simulink library "ammclib_bam_S32K14x"  (R2016a)
settings: Solver=VariableStepAuto  SolverMode=SingleTasking  StartTime=0.0  StopTime=10.0  RelTol=1e-3
undefined symbols (not defined in the file or in its folder): f16A1, f16A2, f16ADCMaxError, f16B0, f16B1, f16B2, f16C1, f16CC1, f16CC1sc, f16CC1sc_D, f16CC1sc_Q, f16CC2, f16CC2sc, f16CC2sc_D, f16CC2sc_Q, f16DerivGain, f16EGain, f16FiltCoef, f16HystOff, f16HystOn, f16IGain, f16IntegGain, f16IntegGainFW, f16IntegGainQ, f16Kd, f16Kq, f16Limit, f16LowerLimit, f16LowerLimit_D, f16LowerLimit_Q, f16LowerLimitFW, f16LowerLimitQ, f16ModIndex, f16OutValOff, f16OutValOn, f16PropGain, f16PropGainFW, f16PropGainQ, f16RampDown, f16RampUp, f16UGain, f16UpperLimit, f16UpperLimit_D, f16UpperLimit_Q, f16UpperLimitFW, f16UpperLimitQ, f16WIGain, f32A1, f32A2, f32ADCMaxError, f32B0, f32B1, f32B2, f32C1, f32CC1, f32CC1sc, f32CC1sc_D, f32CC1sc_Q, f32CC2, f32CC2sc ... (+114)
(part 18 of 22)

== system ammclib_bam_S32K14x/AMCLIB/FLT/AMCLIB_Windmilling_FLT ==
  pUabcIn : Inport  OutDataTypeStr=Bus: SWLIBS_3Syst_FLT  BusOutputAsStruct=on
  AMCLIB_Windmilling_SF : S-Function  FunctionName=AMCLIB_Windmilling_SF_FLT  Parameters=showStates,fltADCMaxError,fltCC1sc,fltCC2sc,fltUpperLimit,fltLowerLimit,fltC1  SFunctionDeploymentMode=off  EnableBusSupport=off
  copyright : Subsystem
      mask Display: text(10,90,'FILE:');text(10,75,'DESRIPTION:');text(10,60,'COPYRIGHT:');text(10,45,'VERSION:');text(10,30,'DATE:')
  copyright2 : Subsystem
      mask Display: text(10,90,'AMCLIB_Windmilling_BAM_FLT.mdl');text(10,75,'PMSM Windmilling');text(10,60,'NXP 2020');text(10,45,'1.0');text(10,30,'28-Mar-2020');
  fltADCMaxError : Ground
  fltAccPI : Ground
  fltAccPI_Out : Terminator
  fltC1 : Ground
  fltCC1sc : Ground
  fltCC2sc : Ground
  fltInErrK1 : Ground
  fltInErrK1_Out : Terminator
  fltInK1 : Ground
  fltInK1_Out : Terminator
  fltLowerLimit : Ground
  fltState : Ground
  fltState_Out : Terminator
  fltUpperLimit : Ground
  u32Lock : Outport
  pPosEst : Outport  Port=2
  pVelocityEst : Outport  Port=3
  wires:
  AMCLIB_Windmilling_SF/7 -> fltInK1_Out/1
  AMCLIB_Windmilling_SF/6 -> fltState_Out/1
  AMCLIB_Windmilling_SF/5 -> fltInErrK1_Out/1
  AMCLIB_Windmilling_SF/4 -> fltAccPI_Out/1
  AMCLIB_Windmilling_SF/3 -> pVelocityEst/1
  AMCLIB_Windmilling_SF/2 -> pPosEst/1
  AMCLIB_Windmilling_SF/1 -> u32Lock/1
  fltInK1/1 -> AMCLIB_Windmilling_SF/11
  fltState/1 -> AMCLIB_Windmilling_SF/10
  fltInErrK1/1 -> AMCLIB_Windmilling_SF/9
  fltAccPI/1 -> AMCLIB_Windmilling_SF/8
  fltC1/1 -> AMCLIB_Windmilling_SF/7
  fltLowerLimit/1 -> AMCLIB_Windmilling_SF/6
  fltUpperLimit/1 -> AMCLIB_Windmilling_SF/5
  fltCC2sc/1 -> AMCLIB_Windmilling_SF/4
  fltCC1sc/1 -> AMCLIB_Windmilling_SF/3
  fltADCMaxError/1 -> AMCLIB_Windmilling_SF/2
  pUabcIn/1 -> AMCLIB_Windmilling_SF/1

== system ammclib_bam_S32K14x/GDFLIB/F16/GDFLIB_FilterFIR_F16 ==
  f16In : Inport  OutDataTypeStr=int16
  GDFLIB_FilterFIR_SF : S-Function  FunctionName=GDFLIB_FilterFIR_SF_F16  Parameters=u16Order,pCoefBuf  SFunctionDeploymentMode=off  EnableBusSupport=off
  copyright : Subsystem
      mask Display: text(10,90,'FILE:');text(10,75,'DESRIPTION:');text(10,60,'COPYRIGHT:');text(10,45,'VERSION:');text(10,30,'DATE:')
  copyright2 : Subsystem
      mask Display: text(10,90,'GDFLIB_FilterFIR_BAM_F16.mdl');text(10,75,'FIR filter.');text(10,60,'NXP 2020');text(10,45,'1.0');text(10,30,'18-Mar-2020');
  f16Out : Outport
  wires:
  GDFLIB_FilterFIR_SF/1 -> f16Out/1
  f16In/1 -> GDFLIB_FilterFIR_SF/1

== system ammclib_bam_S32K14x/GDFLIB/F16/GDFLIB_FilterIIR1_F16 ==
  f16In : Inport  OutDataTypeStr=int16
  GDFLIB_FilterIIR1_SF : S-Function  FunctionName=GDFLIB_FilterIIR1_SF_F16  Parameters=showStates,f16B0,f16B1,f16A1  SFunctionDeploymentMode=off  EnableBusSupport=off
  copyright : Subsystem
      mask Display: text(10,90,'FILE:');text(10,75,'DESRIPTION:');text(10,60,'COPYRIGHT:');text(10,45,'VERSION:');text(10,30,'DATE:')
  copyright2 : Subsystem
      mask Display: text(10,90,'GDFLIB_FilterIIR1_BAM_F16.mdl');text(10,75,'First order IIR filter.');text(10,60,'NXP 2020');text(10,45,'1.0');text(10,30,'18-Mar-2020');
  f16A1 : Ground
  f16B0 : Ground
  f16B1 : Ground
  f16FiltBufferX : Ground
  f16FiltBufferX_Out : Terminator
  f32FiltBufferY : Ground
  f32FiltBufferY_Out : Terminator
  f16Out : Outport
  wires:
  GDFLIB_FilterIIR1_SF/3 -> f32FiltBufferY_Out/1
  GDFLIB_FilterIIR1_SF/2 -> f16FiltBufferX_Out/1
  GDFLIB_FilterIIR1_SF/1 -> f16Out/1
  f32FiltBufferY/1 -> GDFLIB_FilterIIR1_SF/6
  f16FiltBufferX/1 -> GDFLIB_FilterIIR1_SF/5
  f16A1/1 -> GDFLIB_FilterIIR1_SF/4
  f16B1/1 -> GDFLIB_FilterIIR1_SF/3
  f16B0/1 -> GDFLIB_FilterIIR1_SF/2
  f16In/1 -> GDFLIB_FilterIIR1_SF/1

== system ammclib_bam_S32K14x/GDFLIB/F16/GDFLIB_FilterIIR2_F16 ==
  f16In : Inport  OutDataTypeStr=int16
  FilterBufferX1_Out : Terminator
  FilterBufferX2_Out : Terminator
  FilterBufferY1_Out : Terminator
  FilterBufferY2_Out : Terminator
  GDFLIB_FilterIIR2_SF : S-Function  FunctionName=GDFLIB_FilterIIR2_SF_F16  Parameters=showStates,f16B0,f16B1,f16B2,f16A1,f16A2  SFunctionDeploymentMode=off  EnableBusSupport=off
  copyright : Subsystem
      mask Display: text(10,90,'FILE:');text(10,75,'DESRIPTION:');text(10,60,'COPYRIGHT:');text(10,45,'VERSION:');text(10,30,'DATE:')
  copyright2 : Subsystem
      mask Display: text(10,90,'GDFLIB_FilterIIR2_BAM_F16.mdl');text(10,75,'First order IIR filter.');text(10,60,'NXP 2020');text(10,45,'1.0');text(10,30,'18-Mar-2020');
  f16A1 : Ground
  f16A2 : Ground
  f16B0 : Ground
  f16B1 : Ground
  f16B2 : Ground
  f16FiltBufferX1 : Ground
  f16FiltBufferX2 : Ground
  f32FiltBufferY1 : Ground
  f32FiltBufferY2 : Ground
  f16Out : Outport
  wires:
  GDFLIB_FilterIIR2_SF/5 -> FilterBufferY2_Out/1
  GDFLIB_FilterIIR2_SF/4 -> FilterBufferY1_Out/1
  GDFLIB_FilterIIR2_SF/3 -> FilterBufferX2_Out/1
  GDFLIB_FilterIIR2_SF/2 -> FilterBufferX1_Out/1
  GDFLIB_FilterIIR2_SF/1 -> f16Out/1
  f16A2/1 -> GDFLIB_FilterIIR2_SF/10
  f16A1/1 -> GDFLIB_FilterIIR2_SF/9
  f16B2/1 -> GDFLIB_FilterIIR2_SF/8
  f16B1/1 -> GDFLIB_FilterIIR2_SF/7
  f16B0/1 -> GDFLIB_FilterIIR2_SF/6
  f32FiltBufferY2/1 -> GDFLIB_FilterIIR2_SF/5
  f32FiltBufferY1/1 -> GDFLIB_FilterIIR2_SF/4
  f16FiltBufferX2/1 -> GDFLIB_FilterIIR2_SF/3
  f16FiltBufferX1/1 -> GDFLIB_FilterIIR2_SF/2
  f16In/1 -> GDFLIB_FilterIIR2_SF/1

== system ammclib_bam_S32K14x/GDFLIB/F16/GDFLIB_FilterMA_F16 ==
  f16In : Inport  OutDataTypeStr=int16
  f16FilterMAOut_preset : Inport  Port=2  OutDataTypeStr=int16
  Reset : ResetPort  DisableCoverage=on
  GDFLIB_FilterMA_SF : S-Function  FunctionName=GDFLIB_FilterMA_SF_F16  Parameters=showStates,resetStatesEnable,u16NSamples  SFunctionDeploymentMode=off  EnableBusSupport=off
  copyright : Subsystem
      mask Display: text(10,90,'FILE:');text(10,75,'DESRIPTION:');text(10,60,'COPYRIGHT:');text(10,45,'VERSION:');text(10,30,'DATE:')
  copyright2 : Subsystem
      mask Display: text(10,90,'GDFLIB_FilterMA_BAM_F16.mdl');text(10,75,'Exponential moving average filter.');text(10,60,'NXP 2020');text(10,45,'1.0');text(10,30,'28-Mar-2020');
  f32Acc : Ground
  f32Acc_Out : Terminator
  u16NSamples : Ground
  f16Out : Outport
  wires:
  GDFLIB_FilterMA_SF/2 -> f32Acc_Out/1
  GDFLIB_FilterMA_SF/1 -> f16Out/1
  f32Acc/1 -> GDFLIB_FilterMA_SF/4
  u16NSamples/1 -> GDFLIB_FilterMA_SF/3
  f16FilterMAOut_preset/1 -> GDFLIB_FilterMA_SF/2
  f16In/1 -> GDFLIB_FilterMA_SF/1

== system ammclib_bam_S32K14x/GDFLIB/F32/GDFLIB_FilterFIR_F32 ==
  f32In : Inport  OutDataTypeStr=int32
  GDFLIB_FilterFIR_SF : S-Function  FunctionName=GDFLIB_FilterFIR_SF_F32  Parameters=u32Order,pCoefBuf  SFunctionDeploymentMode=off  EnableBusSupport=off
  copyright : Subsystem
      mask Display: text(10,90,'FILE:');text(10,75,'DESRIPTION:');text(10,60,'COPYRIGHT:');text(10,45,'VERSION:');text(10,30,'DATE:')
  copyright2 : Subsystem
      mask Display: text(10,90,'GDFLIB_FilterFIR_BAM_F32.mdl');text(10,75,'FIR filter.');text(10,60,'NXP 2020');text(10,45,'1.0');text(10,30,'18-Mar-2020');
  f32Out : Outport
  wires:
  GDFLIB_FilterFIR_SF/1 -> f32Out/1
  f32In/1 -> GDFLIB_FilterFIR_SF/1

== system ammclib_bam_S32K14x/GDFLIB/F32/GDFLIB_FilterIIR1_F32 ==
  f32In : Inport  OutDataTypeStr=int32
  GDFLIB_FilterIIR1_SF : S-Function  FunctionName=GDFLIB_FilterIIR1_SF_F32  Parameters=showStates,f32B0,f32B1,f32A1  SFunctionDeploymentMode=off  EnableBusSupport=off
  copyright : Subsystem
      mask Display: text(10,90,'FILE:');text(10,75,'DESRIPTION:');text(10,60,'COPYRIGHT:');text(10,45,'VERSION:');text(10,30,'DATE:')
  copyright2 : Subsystem
      mask Display: text(10,90,'GDFLIB_FilterIIR1_BAM_F32.mdl');text(10,75,'First order IIR filter.');text(10,60,'NXP 2020');text(10,45,'1.0');text(10,30,'18-Mar-2020');
  f32A1 : Ground
  f32B0 : Ground
  f32B1 : Ground
  f32FiltBufferX : Ground
  f32FiltBufferX_Out : Terminator
  f32FiltBufferY : Ground
  f32FiltBufferY_Out : Terminator
  f32Out : Outport
  wires:
  GDFLIB_FilterIIR1_SF/3 -> f32FiltBufferY_Out/1
  GDFLIB_FilterIIR1_SF/2 -> f32FiltBufferX_Out/1
  GDFLIB_FilterIIR1_SF/1 -> f32Out/1
  f32FiltBufferY/1 -> GDFLIB_FilterIIR1_SF/6
  f32FiltBufferX/1 -> GDFLIB_FilterIIR1_SF/5
  f32A1/1 -> GDFLIB_FilterIIR1_SF/4
  f32B1/1 -> GDFLIB_FilterIIR1_SF/3
  f32B0/1 -> GDFLIB_FilterIIR1_SF/2
  f32In/1 -> GDFLIB_FilterIIR1_SF/1

== system ammclib_bam_S32K14x/GDFLIB/F32/GDFLIB_FilterIIR2_F32 ==
  f32In : Inport  OutDataTypeStr=int32
  FilterBufferX1_Out : Terminator
  FilterBufferX2_Out : Terminator
  FilterBufferY1_Out : Terminator
  FilterBufferY2_Out : Terminator
  GDFLIB_FilterIIR2_SF : S-Function  FunctionName=GDFLIB_FilterIIR2_SF_F32  Parameters=showStates,f32B0,f32B1,f32B2,f32A1,f32A2  SFunctionDeploymentMode=off  EnableBusSupport=off
  copyright : Subsystem
      mask Display: text(10,90,'FILE:');text(10,75,'DESRIPTION:');text(10,60,'COPYRIGHT:');text(10,45,'VERSION:');text(10,30,'DATE:')
  copyright2 : Subsystem
      mask Display: text(10,90,'GDFLIB_FilterIIR2_BAM_F32.mdl');text(10,75,'First order IIR filter.');text(10,60,'NXP 2020');text(10,45,'1.0');text(10,30,'18-Mar-2020');
  f32A1 : Ground
  f32A2 : Ground
  f32B0 : Ground
  f32B1 : Ground
  f32B2 : Ground
  f32FiltBufferX1 : Ground
  f32FiltBufferX2 : Ground
  f32FiltBufferY1 : Ground
  f32FiltBufferY2 : Ground
  f32Out : Outport
  wires:
  GDFLIB_FilterIIR2_SF/5 -> FilterBufferY2_Out/1
  GDFLIB_FilterIIR2_SF/4 -> FilterBufferY1_Out/1
  GDFLIB_FilterIIR2_SF/3 -> FilterBufferX2_Out/1
  GDFLIB_FilterIIR2_SF/2 -> FilterBufferX1_Out/1
  GDFLIB_FilterIIR2_SF/1 -> f32Out/1
  f32A2/1 -> GDFLIB_FilterIIR2_SF/10
  f32A1/1 -> GDFLIB_FilterIIR2_SF/9
  f32B2/1 -> GDFLIB_FilterIIR2_SF/8
  f32B1/1 -> GDFLIB_FilterIIR2_SF/7
  f32B0/1 -> GDFLIB_FilterIIR2_SF/6
  f32FiltBufferY2/1 -> GDFLIB_FilterIIR2_SF/5
  f32FiltBufferY1/1 -> GDFLIB_FilterIIR2_SF/4
  f32FiltBufferX2/1 -> GDFLIB_FilterIIR2_SF/3
  f32FiltBufferX1/1 -> GDFLIB_FilterIIR2_SF/2
  f32In/1 -> GDFLIB_FilterIIR2_SF/1

== system ammclib_bam_S32K14x/GDFLIB/F32/GDFLIB_FilterMA_F32 ==
  f32In : Inport  OutDataTypeStr=int32
  f32FilterMAOut_preset : Inport  Port=2  OutDataTypeStr=int32
  Reset : ResetPort  DisableCoverage=on
  GDFLIB_FilterMA_SF : S-Function  FunctionName=GDFLIB_FilterMA_SF_F32  Parameters=showStates,resetStatesEnable,u16NSamples  SFunctionDeploymentMode=off  EnableBusSupport=off
  copyright : Subsystem
      mask Display: text(10,90,'FILE:');text(10,75,'DESRIPTION:');text(10,60,'COPYRIGHT:');text(10,45,'VERSION:');text(10,30,'DATE:')
  copyright2 : Subsystem
      mask Display: text(10,90,'GDFLIB_FilterMA_BAM_F32.mdl');text(10,75,'Exponential moving average filter.');text(10,60,'NXP 2020');text(10,45,'1.0');text(10,30,'28-Mar-2020');
  f32Acc : Ground
  f32Acc_Out : Terminator
  u16NSamples : Ground
  f32Out : Outport
  wires:
  GDFLIB_FilterMA_SF/2 -> f32Acc_Out/1
  GDFLIB_FilterMA_SF/1 -> f32Out/1
  f32Acc/1 -> GDFLIB_FilterMA_SF/4
  u16NSamples/1 -> GDFLIB_FilterMA_SF/3
  f32FilterMAOut_preset/1 -> GDFLIB_FilterMA_SF/2
  f32In/1 -> GDFLIB_FilterMA_SF/1

== system ammclib_bam_S32K14x/GDFLIB/FLT/GDFLIB_FilterFIR_FLT ==
  fltIn : Inport  OutDataTypeStr=single
  GDFLIB_FilterFIR_SF : S-Function  FunctionName=GDFLIB_FilterFIR_SF_FLT  Parameters=u32Order,pCoefBuf  SFunctionDeploymentMode=off  EnableBusSupport=off
  copyright : Subsystem
      mask Display: text(10,90,'FILE:');text(10,75,'DESRIPTION:');text(10,60,'COPYRIGHT:');text(10,45,'VERSION:');text(10,30,'DATE:')
  copyright2 : Subsystem
      mask Display: text(10,90,'GDFLIB_FilterFIR_BAM_FLT.mdl');text(10,75,'FIR filter.');text(10,60,'NXP 2020');text(10,45,'1.0');text(10,30,'18-Mar-2020');
  fltOut : Outport
  wires:
  GDFLIB_FilterFIR_SF/1 -> fltOut/1
  fltIn/1 -> GDFLIB_FilterFIR_SF/1

== system ammclib_bam_S32K14x/GDFLIB/FLT/GDFLIB_FilterIIR1_FLT ==
  fltIn : Inport  OutDataTypeStr=single
  GDFLIB_FilterIIR1_SF : S-Function  FunctionName=GDFLIB_FilterIIR1_SF_FLT  Parameters=showStates,fltB0,fltB1,fltA1  SFunctionDeploymentMode=off  EnableBusSupport=off
  copyright : Subsystem
      mask Display: text(10,90,'FILE:');text(10,75,'DESRIPTION:');text(10,60,'COPYRIGHT:');text(10,45,'VERSION:');text(10,30,'DATE:')
  copyright2 : Subsystem
      mask Display: text(10,90,'GDFLIB_FilterIIR1_BAM_FLT.mdl');text(10,75,'First order IIR filter.');text(10,60,'NXP 2020');text(10,45,'1.0');text(10,30,'18-Mar-2020');
  fltA1 : Ground
  fltB0 : Ground
  fltB1 : Ground
  fltFiltBufferX : Ground
  fltFiltBufferX_Out : Terminator
  fltFiltBufferY : Ground
  fltFiltBufferY_Out : Terminator
  fltOut : Outport
  wires:
  GDFLIB_FilterIIR1_SF/3 -> fltFiltBufferY_Out/1
  GDFLIB_FilterIIR1_SF/2 -> fltFiltBufferX_Out/1
  GDFLIB_FilterIIR1_SF/1 -> fltOut/1
  fltFiltBufferY/1 -> GDFLIB_FilterIIR1_SF/6
  fltFiltBufferX/1 -> GDFLIB_FilterIIR1_SF/5
  fltA1/1 -> GDFLIB_FilterIIR1_SF/4
  fltB1/1 -> GDFLIB_FilterIIR1_SF/3
  fltB0/1 -> GDFLIB_FilterIIR1_SF/2
  fltIn/1 -> GDFLIB_FilterIIR1_SF/1

== system ammclib_bam_S32K14x/GDFLIB/FLT/GDFLIB_FilterIIR2_FLT ==
  fltIn : Inport  OutDataTypeStr=single
  FilterBufferX1_Out : Terminator
  FilterBufferX2_Out : Terminator
  FilterBufferY1_Out : Terminator
  FilterBufferY2_Out : Terminator
  GDFLIB_FilterIIR2_SF : S-Function  FunctionName=GDFLIB_FilterIIR2_SF_FLT  Parameters=showStates,fltB0,fltB1,fltB2,fltA1,fltA2  SFunctionDeploymentMode=off  EnableBusSupport=off
  copyright : Subsystem
      mask Display: text(10,90,'FILE:');text(10,75,'DESRIPTION:');text(10,60,'COPYRIGHT:');text(10,45,'VERSION:');text(10,30,'DATE:')
  copyright2 : Subsystem
      mask Display: text(10,90,'GDFLIB_FilterIIR2_BAM_FLT.mdl');text(10,75,'First order IIR filter.');text(10,60,'NXP 2020');text(10,45,'1.0');text(10,30,'18-Mar-2020');
  fltA1 : Ground
  fltA2 : Ground
  fltB0 : Ground
  fltB1 : Ground
  fltB2 : Ground
  fltFiltBufferX1 : Ground
  fltFiltBufferX2 : Ground
  fltFiltBufferY1 : Ground
  fltFiltBufferY2 : Ground
  fltOut : Outport
  wires:
  GDFLIB_FilterIIR2_SF/5 -> FilterBufferY2_Out/1
  GDFLIB_FilterIIR2_SF/4 -> FilterBufferY1_Out/1
  GDFLIB_FilterIIR2_SF/3 -> FilterBufferX2_Out/1
  GDFLIB_FilterIIR2_SF/2 -> FilterBufferX1_Out/1
  GDFLIB_FilterIIR2_SF/1 -> fltOut/1
  fltA2/1 -> GDFLIB_FilterIIR2_SF/10
  fltA1/1 -> GDFLIB_FilterIIR2_SF/9
  fltB2/1 -> GDFLIB_FilterIIR2_SF/8
  fltB1/1 -> GDFLIB_FilterIIR2_SF/7
  fltB0/1 -> GDFLIB_FilterIIR2_SF/6
  fltFiltBufferY2/1 -> GDFLIB_FilterIIR2_SF/5
  fltFiltBufferY1/1 -> GDFLIB_FilterIIR2_SF/4
  fltFiltBufferX2/1 -> GDFLIB_FilterIIR2_SF/3
  fltFiltBufferX1/1 -> GDFLIB_FilterIIR2_SF/2
  fltIn/1 -> GDFLIB_FilterIIR2_SF/1

== system ammclib_bam_S32K14x/GDFLIB/FLT/GDFLIB_FilterMA_FLT ==
  fltIn : Inport  OutDataTypeStr=single
  fltFilterMAOut_preset : Inport  Port=2  OutDataTypeStr=single
  Reset : ResetPort  DisableCoverage=on
  GDFLIB_FilterMA_SF : S-Function  FunctionName=GDFLIB_FilterMA_SF_FLT  Parameters=showStates,resetStatesEnable,fltLambda  SFunctionDeploymentMode=off  EnableBusSupport=off
  copyright : Subsystem
      mask Display: text(10,90,'FILE:');text(10,75,'DESRIPTION:');text(10,60,'COPYRIGHT:');text(10,45,'VERSION:');text(10,30,'DATE:')
  copyright2 : Subsystem
      mask Display: text(10,90,'GDFLIB_FilterMA_BAM_FLT.mdl');text(10,75,'Exponential moving average filter.');text(10,60,'NXP 2020');text(10,45,'1.0');text(10,30,'28-Mar-2020');
  fltAcc : Ground
  fltAcc_Out : Terminator
  fltLambda : Ground
  fltOut : Outport
  wires:
  GDFLIB_FilterMA_SF/2 -> fltAcc_Out/1
  GDFLIB_FilterMA_SF/1 -> fltOut/1
  fltAcc/1 -> GDFLIB_FilterMA_SF/4
  fltLambda/1 -> GDFLIB_FilterMA_SF/3
  fltFilterMAOut_preset/1 -> GDFLIB_FilterMA_SF/2
  fltIn/1 -> GDFLIB_FilterMA_SF/1

== system ammclib_bam_S32K14x/GFLIB/F16/GFLIB_Acos_F16 ==
  f16In : Inport  OutDataTypeStr=int16
  GFLIB_Acos_SF : S-Function  FunctionName=GFLIB_Acos_SF_F16  SFunctionDeploymentMode=off  EnableBusSupport=off
  copyright : Subsystem
      mask Display: text(10,90,'FILE:');text(10,75,'DESRIPTION:');text(10,60,'COPYRIGHT:');text(10,45,'VERSION:');text(10,30,'DATE:')
  copyright2 : Subsystem
      mask Display: text(10,90,'GFLIB_Acos_BAM_F16.mdl');text(10,75,'Inverse cosine function');text(10,60,'NXP 2020');text(10,45,'1.0');text(10,30,'18-Mar-2020');
  f16Out : Outport
  wires:
  GFLIB_Acos_SF/1 -> f16Out/1
  f16In/1 -> GFLIB_Acos_SF/1

== system ammclib_bam_S32K14x/GFLIB/F16/GFLIB_Asin_F16 ==
  f16In : Inport  OutDataTypeStr=int16
  GFLIB_Asin_SF : S-Function  FunctionName=GFLIB_Asin_SF_F16  SFunctionDeploymentMode=off  EnableBusSupport=off
  copyright : Subsystem
      mask Display: text(10,90,'FILE:');text(10,75,'DESRIPTION:');text(10,60,'COPYRIGHT:');text(10,45,'VERSION:');text(10,30,'DATE:')
  copyright2 : Subsystem
      mask Display: text(10,90,'GFLIB_Asin_BAM_F16.mdl');text(10,75,'Inverse sine function');text(10,60,'NXP 2020');text(10,45,'1.0');text(10,30,'18-Mar-2020');
  f16Out : Outport
  wires:
  GFLIB_Asin_SF/1 -> f16Out/1
  f16In/1 -> GFLIB_Asin_SF/1

== system ammclib_bam_S32K14x/GFLIB/F16/GFLIB_AtanYXShifted_F16 ==
  f16InY : Inport  OutDataTypeStr=int16
  f16InX : Inport  Port=2  OutDataTypeStr=int16
  Ky : Inport  Port=3  OutDataTypeStr=int16
  Kx : Inport  Port=4  OutDataTypeStr=int16
  Ny : Inport  Port=5  OutDataTypeStr=int16
  Nx : Inport  Port=6  OutDataTypeStr=int16
  ThetaAdj : Inport  Port=7  OutDataTypeStr=int16
  GFLIB_AtanYXShifted_SF : S-Function  FunctionName=GFLIB_AtanYXShifted_SF_F16  SFunctionDeploymentMode=off  EnableBusSupport=off
  copyright : Subsystem
      mask Display: text(10,90,'FILE:');text(10,75,'DESRIPTION:');text(10,60,'COPYRIGHT:');text(10,45,'VERSION:');text(10,30,'DATE:')
  copyright2 : Subsystem
      mask Display: text(10,90,'GFLIB_AtanYXShifted_BAM_F16.mdl');text(10,75,'Shifted arctangent of two arguments Y/X.');text(10,60,'NXP 2020');text(10,45,'1.0');text(10,30,'18-Mar-2020');
  f16Out : Outport
  wires:
  GFLIB_AtanYXShifted_SF/1 -> f16Out/1
  ThetaAdj/1 -> GFLIB_AtanYXShifted_SF/7
  Nx/1 -> GFLIB_AtanYXShifted_SF/6
  Ny/1 -> GFLIB_AtanYXShifted_SF/5
  Kx/1 -> GFLIB_AtanYXShifted_SF/4
  Ky/1 -> GFLIB_AtanYXShifted_SF/3
  f16InX/1 -> GFLIB_AtanYXShifted_SF/2
  f16InY/1 -> GFLIB_AtanYXShifted_SF/1

== system ammclib_bam_S32K14x/GFLIB/F16/GFLIB_AtanYX_F16 ==
  f16InY : Inport  OutDataTypeStr=int16
  f16InX : Inport  Port=2  OutDataTypeStr=int16
  GFLIB_AtanYX_SF : S-Function  FunctionName=GFLIB_AtanYX_SF_F16  SFunctionDeploymentMode=off  EnableBusSupport=off
  copyright : Subsystem
      mask Display: text(10,90,'FILE:');text(10,75,'DESRIPTION:');text(10,60,'COPYRIGHT:');text(10,45,'VERSION:');text(10,30,'DATE:')
  copyright2 : Subsystem
      mask Display: text(10,90,'GFLIB_AtanYX_BAM_F16.mdl');text(10,75,'Arctangent of two arguments Y/X.');text(10,60,'NXP 2020');text(10,45,'1.0');text(10,30,'18-Mar-2020');
  f16Out : Outport
  wires:
  GFLIB_AtanYX_SF/1 -> f16Out/1
  f16InX/1 -> GFLIB_AtanYX_SF/2
  f16InY/1 -> GFLIB_AtanYX_SF/1

== system ammclib_bam_S32K14x/GFLIB/F16/GFLIB_Atan_F16 ==
  f16In : Inport  OutDataTypeStr=int16
  GFLIB_Atan_SF : S-Function  FunctionName=GFLIB_Atan_SF_F16  SFunctionDeploymentMode=off  EnableBusSupport=off
  copyright : Subsystem
      mask Display: text(10,90,'FILE:');text(10,75,'DESRIPTION:');text(10,60,'COPYRIGHT:');text(10,45,'VERSION:');text(10,30,'DATE:')
  copyright2 : Subsystem
      mask Display: text(10,90,'GFLIB_Atan_BAM_F16.mdl');text(10,75,'Inverse tangent function');text(10,60,'NXP 2020');text(10,45,'1.0');text(10,30,'18-Mar-2020');
  f16Out : Outport
  wires:
  GFLIB_Atan_SF/1 -> f16Out/1
  f16In/1 -> GFLIB_Atan_SF/1

== system ammclib_bam_S32K14x/GFLIB/F16/GFLIB_ControllerPIDpAW_F16 ==
  f16InErr : Inport  OutDataTypeStr=int16
  f16ControllerPIDpAWOut_preset : Inport  Port=2  OutDataTypeStr=int16
  Reset : ResetPort  DisableCoverage=on
  GFLIB_ControllerPIDpAW_SF : S-Function  FunctionName=GFLIB_ControllerPIDpAW_SF_F16  Parameters=showStates,resetStatesEnable,f16PropGain,f16IntegGain,f16DerivGain,f16FiltCoef,s16PropGainShift,s16IntegGainShift,s16DerivGainShift,f16LowerLimit,f16UpperLimit  SFunctionDeploymentMode=off  EnableBusSupport=off
  copyright : Subsystem
      mask Display: text(10,90,'FILE:');text(10,75,'DESRIPTION:');text(10,60,'COPYRIGHT:');text(10,45,'VERSION:');text(10,30,'DATE:')
  copyright2 : Subsystem
      mask Display: text(10,90,'GFLIB_ControllerPIDpAW_BAM_F16.mdl');text(10,75,'Parallel form of a standard PID controller with anti-windup.');text(10,60,'NXP 2020');text(10,45,'1.0');text(10,30,'28-Mar-2020');
  f16DerivGain : Ground
  f16DerivPartK_1 : Ground
  f16DerivPartK_1_Out : Terminator
  f16FiltCoef : Ground
  f16InK_1 : Ground
  f16InK_1_Out : Terminator
  f16IntegGain : Ground
  f16LowerLimit : Ground
  f16PropGain : Ground
  f16UpperLimit : Ground
  f32IntegPartK_1 : Ground
  f32IntegPartK_1_Out : Terminator
  s16DerivGainShift : Ground
  s16IntegGainShift : Ground
  s16PropGainShift : Ground
  f16Out : Outport
  u16LimitFlag : Outport  Port=2
  wires:
  GFLIB_ControllerPIDpAW_SF/5 -> f16InK_1_Out/1
  GFLIB_ControllerPIDpAW_SF/4 -> f16DerivPartK_1_Out/1
  GFLIB_ControllerPIDpAW_SF/3 -> f32IntegPartK_1_Out/1
  GFLIB_ControllerPIDpAW_SF/2 -> u16LimitFlag/1
  GFLIB_ControllerPIDpAW_SF/1 -> f16Out/1
  f16InK_1/1 -> GFLIB_ControllerPIDpAW_SF/14
  f16DerivPartK_1/1 -> GFLIB_ControllerPIDpAW_SF/13
  f32IntegPartK_1/1 -> GFLIB_ControllerPIDpAW_SF/12
  f16UpperLimit/1 -> GFLIB_ControllerPIDpAW_SF/11
  f16LowerLimit/1 -> GFLIB_ControllerPIDpAW_SF/10
  s16DerivGainShift/1 -> GFLIB_ControllerPIDpAW_SF/9
  s16IntegGainShift/1 -> GFLIB_ControllerPIDpAW_SF/8
  s16PropGainShift/1 -> GFLIB_ControllerPIDpAW_SF/7
  f16FiltCoef/1 -> GFLIB_ControllerPIDpAW_SF/6
  f16DerivGain/1 -> GFLIB_ControllerPIDpAW_SF/5
  f16IntegGain/1 -> GFLIB_ControllerPIDpAW_SF/4
  f16PropGain/1 -> GFLIB_ControllerPIDpAW_SF/3
  f16ControllerPIDpAWOut_preset/1 -> GFLIB_ControllerPIDpAW_SF/2
  f16InErr/1 -> GFLIB_ControllerPIDpAW_SF/1

== system ammclib_bam_S32K14x/GFLIB/F16/GFLIB_ControllerPIpAW_F16 ==
  f16InErr : Inport  OutDataTypeStr=int16
  f16ControllerPIpAWOut_preset : Inport  Port=2  OutDataTypeStr=int16
  Reset : ResetPort  DisableCoverage=on
  GFLIB_ControllerPIpAW_SF : S-Function  FunctionName=GFLIB_ControllerPIpAW_SF_F16  Parameters=showStates,resetStatesEnable,f16PropGain,f16IntegGain,s16PropGainShift,s16IntegGainShift,f16LowerLimit,f16UpperLimit  SFunctionDeploymentMode=off  EnableBusSupport=off
  copyright : Subsystem
      mask Display: text(10,90,'FILE:');text(10,75,'DESRIPTION:');text(10,60,'COPYRIGHT:');text(10,45,'VERSION:');text(10,30,'DATE:')
  copyright2 : Subsystem
      mask Display: text(10,90,'GFLIB_ControllerPIpAW_BAM_F16.mdl');text(10,75,'Parallel form of a standard PI controller with anti-windup.');text(10,60,'NXP 2020');text(10,45,'1.0');text(10,30,'28-Mar-2020');
  f16InK_1 : Ground
  f16InK_1_Out : Terminator
  f16IntegGain : Ground
  f16LowerLimit : Ground
  f16PropGain : Ground
  f16UpperLimit : Ground
  f32IntegPartK_1 : Ground
  f32IntegPartK_1_Out : Terminator
  s16IntegGainShift : Ground
  s16PropGainShift : Ground
  f16Out : Outport
  u16LimitFlag : Outport  Port=2
  wires:
  GFLIB_ControllerPIpAW_SF/4 -> f16InK_1_Out/1
  GFLIB_ControllerPIpAW_SF/3 -> f32IntegPartK_1_Out/1
  GFLIB_ControllerPIpAW_SF/2 -> u16LimitFlag/1
  GFLIB_ControllerPIpAW_SF/1 -> f16Out/1
  f16InK_1/1 -> GFLIB_ControllerPIpAW_SF/10
  f32IntegPartK_1/1 -> GFLIB_ControllerPIpAW_SF/9
  f16UpperLimit/1 -> GFLIB_ControllerPIpAW_SF/8
  f16LowerLimit/1 -> GFLIB_ControllerPIpAW_SF/7
  s16IntegGainShift/1 -> GFLIB_ControllerPIpAW_SF/6
  s16PropGainShift/1 -> GFLIB_ControllerPIpAW_SF/5
  f16IntegGain/1 -> GFLIB_ControllerPIpAW_SF/4
  f16PropGain/1 -> GFLIB_ControllerPIpAW_SF/3
  f16ControllerPIpAWOut_preset/1 -> GFLIB_ControllerPIpAW_SF/2
  f16InErr/1 -> GFLIB_ControllerPIpAW_SF/1

== system ammclib_bam_S32K14x/GFLIB/F16/GFLIB_ControllerPIp_F16 ==
  f16InErr : Inport  OutDataTypeStr=int16
  f16ControllerPIpOut_preset : Inport  Port=2  OutDataTypeStr=int16
  Reset : ResetPort  DisableCoverage=on
  GFLIB_ControllerPIp_SF : S-Function  FunctionName=GFLIB_ControllerPIp_SF_F16  Parameters=showStates,resetStatesEnable,f16PropGain,f16IntegGain,s16PropGainShift,s16IntegGainShift  SFunctionDeploymentMode=off  EnableBusSupport=off
  copyright : Subsystem
      mask Display: text(10,90,'FILE:');text(10,75,'DESRIPTION:');text(10,60,'COPYRIGHT:');text(10,45,'VERSION:');text(10,30,'DATE:')
  copyright2 : Subsystem
      mask Display: text(10,90,'GFLIB_ControllerPIp_BAM_F16.mdl');text(10,75,'Parallel form of a standard PI controller without anti-windup.');text(10,60,'NXP 2020');text(10,45,'1.0');text(10,30,'28-Mar-2020');
  f16InK_1 : Ground
  f16InK_1_Out : Terminator
  f16IntegGain : Ground
  f16PropGain : Ground
  f32IntegPartK_1 : Ground
  f32IntegPartK_1_Out : Terminator
  s16IntegGainShift : Ground
  s16PropGainShift : Ground
  f16Out : Outport
  wires:
  GFLIB_ControllerPIp_SF/3 -> f16InK_1_Out/1
  GFLIB_ControllerPIp_SF/2 -> f32IntegPartK_1_Out/1
  GFLIB_ControllerPIp_SF/1 -> f16Out/1
  f16InK_1/1 -> GFLIB_ControllerPIp_SF/8
  f32IntegPartK_1/1 -> GFLIB_ControllerPIp_SF/7
  s16IntegGainShift/1 -> GFLIB_ControllerPIp_SF/6
  s16PropGainShift/1 -> GFLIB_ControllerPIp_SF/5
  f16IntegGain/1 -> GFLIB_ControllerPIp_SF/4
  f16PropGain/1 -> GFLIB_ControllerPIp_SF/3
  f16ControllerPIpOut_preset/1 -> GFLIB_ControllerPIp_SF/2
  f16InErr/1 -> GFLIB_ControllerPIp_SF/1

== system ammclib_bam_S32K14x/GFLIB/F16/GFLIB_ControllerPIrAW_F16 ==
  f16InErr : Inport  OutDataTypeStr=int16
  f16ControllerPIrAWOut_preset : Inport  Port=2  OutDataTypeStr=int16
  Reset : ResetPort  DisableCoverage=on
  GFLIB_ControllerPIrAW_SF : S-Function  FunctionName=GFLIB_ControllerPIrAW_SF_F16  Parameters=showStates,resetStatesEnable,f16UpperLimit,f16LowerLimit,f16CC1sc,f16CC2sc,u16NShift  SFunctionDeploymentMode=off  EnableBusSupport=off
  copyright : Subsystem
      mask Display: text(10,90,'FILE:');text(10,75,'DESRIPTION:');text(10,60,'COPYRIGHT:');text(10,45,'VERSION:');text(10,30,'DATE:')
  copyright2 : Subsystem
      mask Display: text(10,90,'GFLIB_ControllerPIrAW_BAM_F16.mdl');text(10,75,'Recurrent form PI controller with anti-windup.');text(10,60,'NXP 2020');text(10,45,'1.0');text(10,30,'28-Mar-2020');
  f16CC1sc : Ground
  f16CC2sc : Ground
  f16InErrK1 : Ground
  f16InErrK1_Out : Terminator
  f16LowerLimit : Ground
  f16UpperLimit : Ground
  f32Acc : Ground
  f32Acc_Out : Terminator
  u16NShift : Ground
  f16Out : Outport
  wires:
  GFLIB_ControllerPIrAW_SF/3 -> f16InErrK1_Out/1
  GFLIB_ControllerPIrAW_SF/2 -> f32Acc_Out/1
  GFLIB_ControllerPIrAW_SF/1 -> f16Out/1
  u16NShift/1 -> GFLIB_ControllerPIrAW_SF/9
  f16CC2sc/1 -> GFLIB_ControllerPIrAW_SF/8
  f16CC1sc/1 -> GFLIB_ControllerPIrAW_SF/7
  f16InErrK1/1 -> GFLIB_ControllerPIrAW_SF/6
  f32Acc/1 -> GFLIB_ControllerPIrAW_SF/5
  f16LowerLimit/1 -> GFLIB_ControllerPIrAW_SF/4
  f16UpperLimit/1 -> GFLIB_ControllerPIrAW_SF/3
  f16ControllerPIrAWOut_preset/1 -> GFLIB_ControllerPIrAW_SF/2
  f16InErr/1 -> GFLIB_ControllerPIrAW_SF/1

== system ammclib_bam_S32K14x/GFLIB/F16/GFLIB_ControllerPIr_F16 ==
  f16InErr : Inport  OutDataTypeStr=int16
  f16ControllerPIrOut_preset : Inport  Port=2  OutDataTypeStr=int16
  Reset : ResetPort  DisableCoverage=on
  GFLIB_ControllerPIr_SF : S-Function  FunctionName=GFLIB_ControllerPIr_SF_F16  Parameters=showStates,resetStatesEnable,f16CC1,f16CC2,u16NShift  SFunctionDeploymentMode=off  EnableBusSupport=off
  copyright : Subsystem
      mask Display: text(10,90,'FILE:');text(10,75,'DESRIPTION:');text(10,60,'COPYRIGHT:');text(10,45,'VERSION:');text(10,30,'DATE:')
  copyright2 : Subsystem
      mask Display: text(10,90,'GFLIB_ControllerPIr_BAM_F16.mdl');text(10,75,'Recurrent form PI controller without anti-windup.');text(10,60,'NXP 2020');text(10,45,'1.0');text(10,30,'28-Mar-2020');
  f16CC1sc : Ground
  f16CC2sc : Ground
  f16InErrK1 : Ground
  f16InErrK1_Out : Terminator
  f32Acc : Ground
  f32Acc_Out : Terminator
  u16NShift : Ground
  f16Out : Outport
  wires:
  GFLIB_ControllerPIr_SF/3 -> f16InErrK1_Out/1
  GFLIB_ControllerPIr_SF/2 -> f32Acc_Out/1
  GFLIB_ControllerPIr_SF/1 -> f16Out/1
  u16NShift/1 -> GFLIB_ControllerPIr_SF/7
  f16InErrK1/1 -> GFLIB_ControllerPIr_SF/6
  f32Acc/1 -> GFLIB_ControllerPIr_SF/5
  f16CC2sc/1 -> GFLIB_ControllerPIr_SF/4
  f16CC1sc/1 -> GFLIB_ControllerPIr_SF/3
  f16ControllerPIrOut_preset/1 -> GFLIB_ControllerPIr_SF/2
  f16InErr/1 -> GFLIB_ControllerPIr_SF/1

== system ammclib_bam_S32K14x/GFLIB/F16/GFLIB_Cos_F16 ==
  f16In : Inport  OutDataTypeStr=int16
  GFLIB_Cos_SF : S-Function  FunctionName=GFLIB_Cos_SF_F16  SFunctionDeploymentMode=off  EnableBusSupport=off
  copyright : Subsystem
      mask Display: text(10,90,'FILE:');text(10,75,'DESRIPTION:');text(10,60,'COPYRIGHT:');text(10,45,'VERSION:');text(10,30,'DATE:')
  copyright2 : Subsystem
      mask Display: text(10,90,'GFLIB_Cos_BAM_F16.mdl');text(10,75,'Cosine function');text(10,60,'NXP 2020');text(10,45,'1.0');text(10,30,'18-Mar-2020');
  f16Out : Outport
  wires:
  GFLIB_Cos_SF/1 -> f16Out/1
  f16In/1 -> GFLIB_Cos_SF/1

== system ammclib_bam_S32K14x/GFLIB/F16/GFLIB_Hyst_F16 ==
  f16In : Inport  OutDataTypeStr=int16
  GFLIB_Hyst_SF : S-Function  FunctionName=GFLIB_Hyst_SF_F16  Parameters=showStates,f16HystOn,f16HystOff,f16OutValOn,f16OutValOff  SFunctionDeploymentMode=off  EnableBusSupport=off
  copyright : Subsystem
      mask Display: text(10,90,'FILE:');text(10,75,'DESRIPTION:');text(10,60,'COPYRIGHT:');text(10,45,'VERSION:');text(10,30,'DATE:')
  copyright2 : Subsystem
      mask Display: text(10,90,'GFLIB_Hyst_BAM_F16.mdl');text(10,75,'Hysteresis function.');text(10,60,'NXP 2020');text(10,45,'1.0');text(10,30,'18-Mar-2020');
  f16HystOff : Ground
  f16HystOn : Ground
  f16OutState : Ground
  f16OutState_Out : Terminator
  f16OutValOff : Ground
  f16OutValOn : Ground
  f16Out : Outport
  wires:
  GFLIB_Hyst_SF/2 -> f16OutState_Out/1
  GFLIB_Hyst_SF/1 -> f16Out/1
  f16OutState/1 -> GFLIB_Hyst_SF/6
  f16OutValOff/1 -> GFLIB_Hyst_SF/5
  f16OutValOn/1 -> GFLIB_Hyst_SF/4
  f16HystOff/1 -> GFLIB_Hyst_SF/3
  f16HystOn/1 -> GFLIB_Hyst_SF/2
  f16In/1 -> GFLIB_Hyst_SF/1

== system ammclib_bam_S32K14x/GFLIB/F16/GFLIB_IntegratorTR_F16 ==
  f16In : Inport  OutDataTypeStr=int16
  f16IntegratorTROut_preset : Inport  Port=2  OutDataTypeStr=int16
  Reset : ResetPort  DisableCoverage=on
  GFLIB_IntegratorTR_SF : S-Function  FunctionName=GFLIB_IntegratorTR_SF_F16  Parameters=showStates,resetStatesEnable,f16C1,u16NShift  SFunctionDeploymentMode=off  EnableBusSupport=off
  copyright : Subsystem
      mask Display: text(10,90,'FILE:');text(10,75,'DESRIPTION:');text(10,60,'COPYRIGHT:');text(10,45,'VERSION:');text(10,30,'DATE:')
  copyright2 : Subsystem
      mask Display: text(10,90,'GFLIB_IntegratorTR_BAM_F16.mdl');text(10,75,'Discrete integrator transformed from a linear model using Billinear (trapezoidal) transformation.');text(10,60,'NXP 2020');text(10,45,'1.0');text(10,30,'28-Mar-2020');
  f16C1 : Ground
  f16InK1 : Ground
  f16InK1_Out : Terminator
  f32State : Ground
  f32State_Out : Terminator
  u16NShift : Ground
  f16Out : Outport
  wires:
  GFLIB_IntegratorTR_SF/3 -> f16InK1_Out/1
  GFLIB_IntegratorTR_SF/2 -> f32State_Out/1
  GFLIB_IntegratorTR_SF/1 -> f16Out/1
  f16InK1/1 -> GFLIB_IntegratorTR_SF/6
  f32State/1 -> GFLIB_IntegratorTR_SF/5
  u16NShift/1 -> GFLIB_IntegratorTR_SF/4
  f16C1/1 -> GFLIB_IntegratorTR_SF/3
  f16IntegratorTROut_preset/1 -> GFLIB_IntegratorTR_SF/2
  f16In/1 -> GFLIB_IntegratorTR_SF/1

== system ammclib_bam_S32K14x/GFLIB/F16/GFLIB_Limit_F16 ==
  f16In : Inport  OutDataTypeStr=int16
  GFLIB_Limit_SF : S-Function  FunctionName=GFLIB_Limit_SF_F16  Parameters=showStates,f16LowerLimit,f16UpperLimit  SFunctionDeploymentMode=off  EnableBusSupport=off
  copyright : Subsystem
      mask Display: text(10,90,'FILE:');text(10,75,'DESRIPTION:');text(10,60,'COPYRIGHT:');text(10,45,'VERSION:');text(10,30,'DATE:')
  copyright2 : Subsystem
      mask Display: text(10,90,'GFLIB_Limit_BAM_F16.mdl');text(10,75,'Limit function.');text(10,60,'NXP 2020');text(10,45,'1.0');text(10,30,'23-Mar-2020');
  f16LowerLimit : Ground
  f16UpperLimit : Ground
  f16Out : Outport
  wires:
  GFLIB_Limit_SF/1 -> f16Out/1
  f16UpperLimit/1 -> GFLIB_Limit_SF/3
  f16LowerLimit/1 -> GFLIB_Limit_SF/2
  f16In/1 -> GFLIB_Limit_SF/1

== system ammclib_bam_S32K14x/GFLIB/F16/GFLIB_LowerLimit_F16 ==
  f16In : Inport  OutDataTypeStr=int16
  GFLIB_LowerLimit_SF : S-Function  FunctionName=GFLIB_LowerLimit_SF_F16  Parameters=showStates,f16LowerLimit  SFunctionDeploymentMode=off  EnableBusSupport=off
  copyright : Subsystem
      mask Display: text(10,90,'FILE:');text(10,75,'DESRIPTION:');text(10,60,'COPYRIGHT:');text(10,45,'VERSION:');text(10,30,'DATE:')
  copyright2 : Subsystem
      mask Display: text(10,90,'GFLIB_LowerLimit_BAM_F16.mdl');text(10,75,'Lower limit function.');text(10,60,'NXP 2020');text(10,45,'1.0');text(10,30,'18-Mar-2020');
  f16LowerLimit : Ground
  f16Out : Outport
  wires:
  GFLIB_LowerLimit_SF/1 -> f16Out/1
  f16LowerLimit/1 -> GFLIB_LowerLimit_SF/2
  f16In/1 -> GFLIB_LowerLimit_SF/1

== system ammclib_bam_S32K14x/GFLIB/F16/GFLIB_Lut1D_F16 ==
  f16In : Inport  OutDataTypeStr=int16
  u16ShamOffset : Inport  Port=2  OutDataTypeStr=uint16
  GFLIB_Lut1D_SF : S-Function  FunctionName=GFLIB_Lut1D_SF_F16  Parameters=pf16Table,s16MidIdx  SFunctionDeploymentMode=off  EnableBusSupport=off
  copyright : Subsystem
      mask Display: text(10,90,'FILE:');text(10,75,'DESRIPTION:');text(10,60,'COPYRIGHT:');text(10,45,'VERSION:');text(10,30,'DATE:')
  copyright2 : Subsystem
      mask Display: text(10,90,'GFLIB_Lut1D_BAM_F16.mdl');text(10,75,'One dimensional lookup table function');text(10,60,'NXP 2020');text(10,45,'1.0');text(10,30,'23-Mar-2020');
  f16Out : Outport
  wires:
  GFLIB_Lut1D_SF/1 -> f16Out/1
  u16ShamOffset/1 -> GFLIB_Lut1D_SF/2
  f16In/1 -> GFLIB_Lut1D_SF/1

== system ammclib_bam_S32K14x/GFLIB/F16/GFLIB_Lut2D_F16 ==
  f16In1 : Inport  OutDataTypeStr=int16
  f16In2 : Inport  Port=2  OutDataTypeStr=int16
  u16ShamOffset1 : Inport  Port=3  OutDataTypeStr=uint16
  u16ShamOffset2 : Inport  Port=4  OutDataTypeStr=uint16
  GFLIB_Lut2D_SF : S-Function  FunctionName=GFLIB_Lut2D_SF_F16  Parameters=pf16Table,s16MidIdx  SFunctionDeploymentMode=off  EnableBusSupport=off
  copyright : Subsystem
      mask Display: text(10,90,'FILE:');text(10,75,'DESRIPTION:');text(10,60,'COPYRIGHT:');text(10,45,'VERSION:');text(10,30,'DATE:')
  copyright2 : Subsystem
      mask Display: text(10,90,'GFLIB_Lut2D_BAM_F16.mdl');text(10,75,'Two dimensional lookup table function');text(10,60,'NXP 2020');text(10,45,'1.0');text(10,30,'23-Mar-2020');
  f16Out : Outport
  wires:
  GFLIB_Lut2D_SF/1 -> f16Out/1
  u16ShamOffset2/1 -> GFLIB_Lut2D_SF/4
  u16ShamOffset1/1 -> GFLIB_Lut2D_SF/3
  f16In2/1 -> GFLIB_Lut2D_SF/2
  f16In1/1 -> GFLIB_Lut2D_SF/1

== system ammclib_bam_S32K14x/GFLIB/F16/GFLIB_Ramp_F16 ==
  f16In : Inport  OutDataTypeStr=int16
  GFLIB_Ramp_SF : S-Function  FunctionName=GFLIB_Ramp_SF_F16  Parameters=showStates,f16RampUp,f16RampDown  SFunctionDeploymentMode=off  EnableBusSupport=off
  copyright : Subsystem
      mask Display: text(10,90,'FILE:');text(10,75,'DESRIPTION:');text(10,60,'COPYRIGHT:');text(10,45,'VERSION:');text(10,30,'DATE:')
  copyright2 : Subsystem
      mask Display: text(10,90,'GFLIB_Ramp_BAM_F16.mdl');text(10,75,'Rate of change limiter - ramp function.');text(10,60,'NXP 2020');text(10,45,'1.0');text(10,30,'18-Mar-2020');
  f16RampDown : Ground
  f16RampUp : Ground
  f16State : Ground
  f16State_Out : Terminator
  f16Out : Outport
  wires:
  GFLIB_Ramp_SF/2 -> f16State_Out/1
  GFLIB_Ramp_SF/1 -> f16Out/1
  f16RampDown/1 -> GFLIB_Ramp_SF/4
  f16RampUp/1 -> GFLIB_Ramp_SF/3
  f16State/1 -> GFLIB_Ramp_SF/2
  f16In/1 -> GFLIB_Ramp_SF/1

== system ammclib_bam_S32K14x/GFLIB/F16/GFLIB_Sign_F16 ==
  f16In : Inport  OutDataTypeStr=int16
  GFLIB_Sign_SF : S-Function  FunctionName=GFLIB_Sign_SF_F16  SFunctionDeploymentMode=off  EnableBusSupport=off
  copyright : Subsystem
      mask Display: text(10,90,'FILE:');text(10,75,'DESRIPTION:');text(10,60,'COPYRIGHT:');text(10,45,'VERSION:');text(10,30,'DATE:')
  copyright2 : Subsystem
      mask Display: text(10,90,'GFLIB_Sign_BAM_F16.mdl');text(10,75,'Sign function.');text(10,60,'NXP 2020');text(10,45,'1.0');text(10,30,'18-Mar-2020');
  f16Out : Outport
  wires:
  GFLIB_Sign_SF/1 -> f16Out/1
  f16In/1 -> GFLIB_Sign_SF/1

== system ammclib_bam_S32K14x/GFLIB/F16/GFLIB_SinCos_F16 ==
  f16In : Inport  OutDataTypeStr=int16
  GFLIB_SinCos_SF : S-Function  FunctionName=GFLIB_SinCos_SF_F16  SFunctionDeploymentMode=off  EnableBusSupport=off
  copyright : Subsystem
      mask Display: text(10,90,'FILE:');text(10,75,'DESRIPTION:');text(10,60,'COPYRIGHT:');text(10,45,'VERSION:');text(10,30,'DATE:')
  copyright2 : Subsystem
      mask Display: text(10,90,'GFLIB_SinCos_BAM_F16.mdl');text(10,75,'Sine and cosine of the same argument');text(10,60,'NXP 2020');text(10,45,'1.0');text(10,30,'18-Mar-2020');
  pOut : Outport
  wires:
  GFLIB_SinCos_SF/1 -> pOut/1
  f16In/1 -> GFLIB_SinCos_SF/1

== system ammclib_bam_S32K14x/GFLIB/F16/GFLIB_Sin_F16 ==
  f16In : Inport  OutDataTypeStr=int16
  GFLIB_Sin_SF : S-Function  FunctionName=GFLIB_Sin_SF_F16  SFunctionDeploymentMode=off  EnableBusSupport=off
  copyright : Subsystem
      mask Display: text(10,90,'FILE:');text(10,75,'DESRIPTION:');text(10,60,'COPYRIGHT:');text(10,45,'VERSION:');text(10,30,'DATE:')
  copyright2 : Subsystem
      mask Display: text(10,90,'GFLIB_Sin_BAM_F16.mdl');text(10,75,'Sine function');text(10,60,'NXP 2020');text(10,45,'1.0');text(10,30,'18-Mar-2020');
  f16Out : Outport
  wires:
  GFLIB_Sin_SF/1 -> f16Out/1
  f16In/1 -> GFLIB_Sin_SF/1

== system ammclib_bam_S32K14x/GFLIB/F16/GFLIB_Sqrt_F16 ==
  f16In : Inport  OutDataTypeStr=int16
  GFLIB_Sqrt_SF : S-Function  FunctionName=GFLIB_Sqrt_SF_F16  SFunctionDeploymentMode=off  EnableBusSupport=off
  copyright : Subsystem
      mask Display: text(10,90,'FILE:');text(10,75,'DESRIPTION:');text(10,60,'COPYRIGHT:');text(10,45,'VERSION:');text(10,30,'DATE:')
  copyright2 : Subsystem
      mask Display: text(10,90,'GFLIB_Sqrt_BAM_F16.mdl');text(10,75,'Square root approximation.');text(10,60,'NXP 2020');text(10,45,'1.0');text(10,30,'18-Mar-2020');
  f16Out : Outport
  wires:
  GFLIB_Sqrt_SF/1 -> f16Out/1
  f16In/1 -> GFLIB_Sqrt_SF/1

== system ammclib_bam_S32K14x/GFLIB/F16/GFLIB_Tan_F16 ==
  f16In : Inport  OutDataTypeStr=int16
  GFLIB_Tan_SF : S-Function  FunctionName=GFLIB_Tan_SF_F16  SFunctionDeploymentMode=off  EnableBusSupport=off
  copyright : Subsystem
      mask Display: text(10,90,'FILE:');text(10,75,'DESRIPTION:');text(10,60,'COPYRIGHT:');text(10,45,'VERSION:');text(10,30,'DATE:')
  copyright2 : Subsystem
      mask Display: text(10,90,'GFLIB_Tan_BAM_F16.mdl');text(10,75,'Trigonometric tangent function');text(10,60,'NXP 2020');text(10,45,'1.0');text(10,30,'18-Mar-2020');
  f16Out : Outport
  wires:
  GFLIB_Tan_SF/1 -> f16Out/1
  f16In/1 -> GFLIB_Tan_SF/1

== system ammclib_bam_S32K14x/GFLIB/F16/GFLIB_UpperLimit_F16 ==
  f16In : Inport  OutDataTypeStr=int16
  GFLIB_UpperLimit_SF : S-Function  FunctionName=GFLIB_UpperLimit_SF_F16  Parameters=showStates,f16UpperLimit  SFunctionDeploymentMode=off  EnableBusSupport=off
  copyright : Subsystem
      mask Display: text(10,90,'FILE:');text(10,75,'DESRIPTION:');text(10,60,'COPYRIGHT:');text(10,45,'VERSION:');text(10,30,'DATE:')
  copyright2 : Subsystem
      mask Display: text(10,90,'GFLIB_UpperLimit_BAM_F16.mdl');text(10,75,'Upper limit function.');text(10,60,'NXP 2020');text(10,45,'1.0');text(10,30,'23-Mar-2020');
  f16UpperLimit : Ground
  f16Out : Outport
  wires:
  GFLIB_UpperLimit_SF/1 -> f16Out/1
  f16UpperLimit/1 -> GFLIB_UpperLimit_SF/2
  f16In/1 -> GFLIB_UpperLimit_SF/1

== system ammclib_bam_S32K14x/GFLIB/F16/GFLIB_VMin_F16 ==
  pIn : Inport  OutDataTypeStr=int16
  GFLIB_VMin_SF : S-Function  FunctionName=GFLIB_VMin_SF_F16  SFunctionDeploymentMode=off  EnableBusSupport=off
  copyright : Subsystem
      mask Display: text(10,90,'FILE:');text(10,75,'DESRIPTION:');text(10,60,'COPYRIGHT:');text(10,45,'VERSION:');text(10,30,'DATE:')
  copyright2 : Subsystem
      mask Display: text(10,90,'GFLIB_VMin_BAM_F16.mdl');text(10,75,'Vector minimum');text(10,60,'NXP 2020');text(10,45,'1.0');text(10,30,'18-Mar-2020');
  IndexOfMinimum : Outport
  wires:
  GFLIB_VMin_SF/1 -> IndexOfMinimum/1
  pIn/1 -> GFLIB_VMin_SF/1

== system ammclib_bam_S32K14x/GFLIB/F16/GFLIB_VectorLimit_F16 ==
  pIn : Inport  OutDataTypeStr=Bus: SWLIBS_2Syst_F16  BusOutputAsStruct=on
  GFLIB_VectorLimit_SF : S-Function  FunctionName=GFLIB_VectorLimit_SF_F16  Parameters=showStates,f16Limit  SFunctionDeploymentMode=off  EnableBusSupport=off
  copyright : Subsystem
      mask Display: text(10,90,'FILE:');text(10,75,'DESRIPTION:');text(10,60,'COPYRIGHT:');text(10,45,'VERSION:');text(10,30,'DATE:')
  copyright2 : Subsystem
      mask Display: text(10,90,'GFLIB_VectorLimit_BAM_F16.mdl');text(10,75,'Vector Limit function.');text(10,60,'NXP 2020');text(10,45,'1.0');text(10,30,'18-Mar-2020');
  f16Limit : Ground
  bFlag : Outport
  pOut : Outport  Port=2
  wires:
  GFLIB_VectorLimit_SF/2 -> pOut/1
  GFLIB_VectorLimit_SF/1 -> bFlag/1
  f16Limit/1 -> GFLIB_VectorLimit_SF/2
  pIn/1 -> GFLIB_VectorLimit_SF/1

== system ammclib_bam_S32K14x/GFLIB/F32/GFLIB_Acos_F32 ==
  f32In : Inport  OutDataTypeStr=int32
  GFLIB_Acos_SF : S-Function  FunctionName=GFLIB_Acos_SF_F32  SFunctionDeploymentMode=off  EnableBusSupport=off
  copyright : Subsystem
      mask Display: text(10,90,'FILE:');text(10,75,'DESRIPTION:');text(10,60,'COPYRIGHT:');text(10,45,'VERSION:');text(10,30,'DATE:')
  copyright2 : Subsystem
      mask Display: text(10,90,'GFLIB_Acos_BAM_F32.mdl');text(10,75,'Inverse cosine function');text(10,60,'NXP 2020');text(10,45,'1.0');text(10,30,'18-Mar-2020');
  f32Out : Outport
  wires:
  GFLIB_Acos_SF/1 -> f32Out/1
  f32In/1 -> GFLIB_Acos_SF/1

== system ammclib_bam_S32K14x/GFLIB/F32/GFLIB_Asin_F32 ==
  f32In : Inport  OutDataTypeStr=int32
  GFLIB_Asin_SF : S-Function  FunctionName=GFLIB_Asin_SF_F32  SFunctionDeploymentMode=off  EnableBusSupport=off
  copyright : Subsystem
      mask Display: text(10,90,'FILE:');text(10,75,'DESRIPTION:');text(10,60,'COPYRIGHT:');text(10,45,'VERSION:');text(10,30,'DATE:')
  copyright2 : Subsystem
      mask Display: text(10,90,'GFLIB_Asin_BAM_F32.mdl');text(10,75,'Inverse sine function');text(10,60,'NXP 2020');text(10,45,'1.0');text(10,30,'18-Mar-2020');
  f32Out : Outport
  wires:
  GFLIB_Asin_SF/1 -> f32Out/1
  f32In/1 -> GFLIB_Asin_SF/1

== system ammclib_bam_S32K14x/GFLIB/F32/GFLIB_AtanYXShifted_F32 ==
  f32InY : Inport  OutDataTypeStr=int32
  f32InX : Inport  Port=2  OutDataTypeStr=int32
  Ky : Inport  Port=3  OutDataTypeStr=int32
  Kx : Inport  Port=4  OutDataTypeStr=int32
  Ny : Inport  Port=5  OutDataTypeStr=int32
  Nx : Inport  Port=6  OutDataTypeStr=int32
  ThetaAdj : Inport  Port=7  OutDataTypeStr=int32
  GFLIB_AtanYXShifted_SF : S-Function  FunctionName=GFLIB_AtanYXShifted_SF_F32  SFunctionDeploymentMode=off  EnableBusSupport=off
  copyright : Subsystem
      mask Display: text(10,90,'FILE:');text(10,75,'DESRIPTION:');text(10,60,'COPYRIGHT:');text(10,45,'VERSION:');text(10,30,'DATE:')
  copyright2 : Subsystem
      mask Display: text(10,90,'GFLIB_AtanYXShifted_BAM_F32.mdl');text(10,75,'Shifted arctangent of two arguments Y/X.');text(10,60,'NXP 2020');text(10,45,'1.0');text(10,30,'18-Mar-2020');
  f32Out : Outport
  wires:
  GFLIB_AtanYXShifted_SF/1 -> f32Out/1
  ThetaAdj/1 -> GFLIB_AtanYXShifted_SF/7
  Nx/1 -> GFLIB_AtanYXShifted_SF/6
  Ny/1 -> GFLIB_AtanYXShifted_SF/5
  Kx/1 -> GFLIB_AtanYXShifted_SF/4
  Ky/1 -> GFLIB_AtanYXShifted_SF/3
  f32InX/1 -> GFLIB_AtanYXShifted_SF/2
  f32InY/1 -> GFLIB_AtanYXShifted_SF/1

== system ammclib_bam_S32K14x/GFLIB/F32/GFLIB_AtanYX_F32 ==
  f32InY : Inport  OutDataTypeStr=int32
  f32InX : Inport  Port=2  OutDataTypeStr=int32
  GFLIB_AtanYX_SF : S-Function  FunctionName=GFLIB_AtanYX_SF_F32  SFunctionDeploymentMode=off  EnableBusSupport=off
  copyright : Subsystem
      mask Display: text(10,90,'FILE:');text(10,75,'DESRIPTION:');text(10,60,'COPYRIGHT:');text(10,45,'VERSION:');text(10,30,'DATE:')
  copyright2 : Subsystem
      mask Display: text(10,90,'GFLIB_AtanYX_BAM_F32.mdl');text(10,75,'Arctangent of two arguments Y/X.');text(10,60,'NXP 2020');text(10,45,'1.0');text(10,30,'18-Mar-2020');
  f32Out : Outport
  wires:
  GFLIB_AtanYX_SF/1 -> f32Out/1
  f32InX/1 -> GFLIB_AtanYX_SF/2
  f32InY/1 -> GFLIB_AtanYX_SF/1

== system ammclib_bam_S32K14x/GFLIB/F32/GFLIB_Atan_F32 ==
  f32In : Inport  OutDataTypeStr=int32
  GFLIB_Atan_SF : S-Function  FunctionName=GFLIB_Atan_SF_F32  SFunctionDeploymentMode=off  EnableBusSupport=off
  copyright : Subsystem
      mask Display: text(10,90,'FILE:');text(10,75,'DESRIPTION:');text(10,60,'COPYRIGHT:');text(10,45,'VERSION:');text(10,30,'DATE:')
  copyright2 : Subsystem
      mask Display: text(10,90,'GFLIB_Atan_BAM_F32.mdl');text(10,75,'Inverse tangent function');text(10,60,'NXP 2020');text(10,45,'1.0');text(10,30,'18-Mar-2020');
  f32Out : Outport
  wires:
  GFLIB_Atan_SF/1 -> f32Out/1
  f32In/1 -> GFLIB_Atan_SF/1

== system ammclib_bam_S32K14x/GFLIB/F32/GFLIB_ControllerPIDpAW_F32 ==
  f32InErr : Inport  OutDataTypeStr=int32
  f32ControllerPIDpAWOut_preset : Inport  Port=2  OutDataTypeStr=int32
  Reset : ResetPort  DisableCoverage=on
  GFLIB_ControllerPIDpAW_SF : S-Function  FunctionName=GFLIB_ControllerPIDpAW_SF_F32  Parameters=showStates,resetStatesEnable,f32PropGain,f32IntegGain,f32DerivGain,f32FiltCoef,s16PropGainShift,s16IntegGainShift,s16DerivGainShift,f32LowerLimit,f32UpperLimit  SFunctionDeploymentMode=off  EnableBusSupport=off
  copyright : Subsystem
      mask Display: text(10,90,'FILE:');text(10,75,'DESRIPTION:');text(10,60,'COPYRIGHT:');text(10,45,'VERSION:');text(10,30,'DATE:')
  copyright2 : Subsystem
      mask Display: text(10,90,'GFLIB_ControllerPIDpAW_BAM_F32.mdl');text(10,75,'Parallel form of a standard PID controller with anti-windup.');text(10,60,'NXP 2020');text(10,45,'1.0');text(10,30,'28-Mar-2020');
  f32DerivGain : Ground
  f32DerivPartK_1 : Ground
  f32DerivPartK_1_Out : Terminator
  f32FiltCoef : Ground
  f32InK_1 : Ground
  f32InK_1_Out : Terminator
  f32IntegGain : Ground
  f32IntegPartK_1 : Ground
  f32IntegPartK_1_Out : Terminator
  f32LowerLimit : Ground
  f32PropGain : Ground
  f32UpperLimit : Ground
  s16DerivGainShift : Ground
  s16IntegGainShift : Ground
  s16PropGainShift : Ground
  f32Out : Outport
  u16LimitFlag : Outport  Port=2
  wires:
  GFLIB_ControllerPIDpAW_SF/5 -> f32InK_1_Out/1
  GFLIB_ControllerPIDpAW_SF/4 -> f32DerivPartK_1_Out/1
  GFLIB_ControllerPIDpAW_SF/3 -> f32IntegPartK_1_Out/1
  GFLIB_ControllerPIDpAW_SF/2 -> u16LimitFlag/1
  GFLIB_ControllerPIDpAW_SF/1 -> f32Out/1
  f32InK_1/1 -> GFLIB_ControllerPIDpAW_SF/14
  f32DerivPartK_1/1 -> GFLIB_ControllerPIDpAW_SF/13
  f32IntegPartK_1/1 -> GFLIB_ControllerPIDpAW_SF/12
  f32UpperLimit/1 -> GFLIB_ControllerPIDpAW_SF/11
  f32LowerLimit/1 -> GFLIB_ControllerPIDpAW_SF/10
  s16DerivGainShift/1 -> GFLIB_ControllerPIDpAW_SF/9
  s16IntegGainShift/1 -> GFLIB_ControllerPIDpAW_SF/8
  s16PropGainShift/1 -> GFLIB_ControllerPIDpAW_SF/7
  f32FiltCoef/1 -> GFLIB_ControllerPIDpAW_SF/6
  f32DerivGain/1 -> GFLIB_ControllerPIDpAW_SF/5
  f32IntegGain/1 -> GFLIB_ControllerPIDpAW_SF/4
  f32PropGain/1 -> GFLIB_ControllerPIDpAW_SF/3
  f32ControllerPIDpAWOut_preset/1 -> GFLIB_ControllerPIDpAW_SF/2
  f32InErr/1 -> GFLIB_ControllerPIDpAW_SF/1
